simulink model "lane_keeping_MPC"  (R2020a)
settings: Solver=FixedStepAuto  StartTime=0.0  StopTime=13  FixedStep=.01  RelTol=1e-3
libraries: simulink x2, mpcadaslib x1
settings Model: EnablePacing=on  Creator=Jamie  LastModifiedBy=Jamie

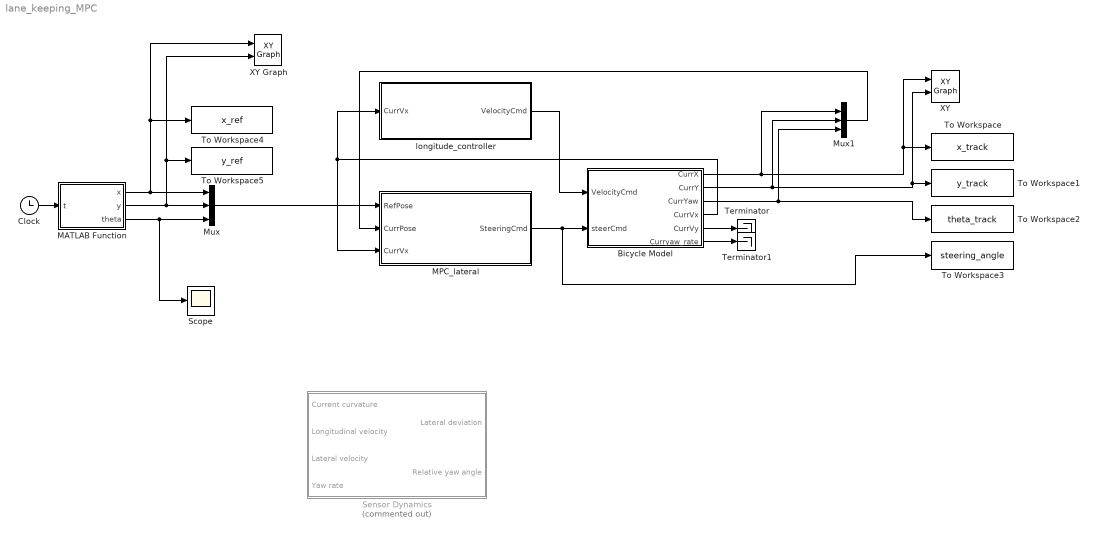
== system lane_keeping_MPC ==
  Bicycle Model : Subsystem
  Clock : Clock
  MATLAB Function : MATLAB Function  TreatAsAtomicUnit=on
  MPC_lateral : Subsystem
  Mux : Mux  Inputs=3
  Mux1 : Mux  Inputs=3
  Scope : Scope
  Sensor Dynamics : Subsystem  Commented=on
  Terminator : Terminator
  Terminator1 : Terminator
  To Workspace : ToWorkspace  VariableName=x_track  SampleTime=-1
      settings: Save2DSignal=2-D array (concatenate along first dimension)
  To Workspace1 : ToWorkspace  VariableName=y_track  SampleTime=-1
      settings: Save2DSignal=2-D array (concatenate along first dimension)
  To Workspace2 : ToWorkspace  VariableName=theta_track  SampleTime=-1
      settings: Save2DSignal=2-D array (concatenate along first dimension)
  To Workspace3 : ToWorkspace  VariableName=steering_angle  SampleTime=-1
      settings: Save2DSignal=2-D array (concatenate along first dimension)
  To Workspace4 : ToWorkspace  VariableName=x_ref  SampleTime=-1
      settings: Save2DSignal=2-D array (concatenate along first dimension)
  To Workspace5 : ToWorkspace  VariableName=y_ref  SampleTime=-1
      settings: Save2DSignal=2-D array (concatenate along first dimension)
  XY : simulink/Sinks/XY Graph  xmin=-10  xmax=10  ymin=-5  ymax=5  st=-1
  XY Graph : simulink/Sinks/XY Graph  xmin=-1  xmax=1  ymin=-1  ymax=1  st=-1
  longitude_controller : Subsystem
  wires:
  Clock/1 -> MATLAB Function/1(t)
  MATLAB Function/1(x) -> Mux/1, XY Graph/1, To Workspace4/1
  MATLAB Function/2(y) -> XY Graph/2, To Workspace5/1, Mux/2
  MATLAB Function/3(theta) -> Scope/1, Mux/3
  MPC_lateral/1(SteeringCmd) -> To Workspace3/1, Bicycle Model/2(steerCmd)
  Bicycle Model/3(CurrYaw) -> To Workspace2/1, Mux1/3
  Bicycle Model/1(CurrX) -> XY/1, To Workspace/1, Mux1/1
  Bicycle Model/2(CurrY) -> XY/2, To Workspace1/1, Mux1/2
  Mux1/1 -> MPC_lateral/2(CurrPose)
  Mux/1 -> MPC_lateral/1(RefPose)
  longitude_controller/1(VelocityCmd) -> Bicycle Model/1(VelocityCmd)
  Bicycle Model/4(CurrVx) -> MPC_lateral/3(CurrVx), longitude_controller/1(CurrVx)
  Bicycle Model/5(CurrVy) -> Terminator/1
  Bicycle Model/6(Curryaw_rate) -> Terminator1/1

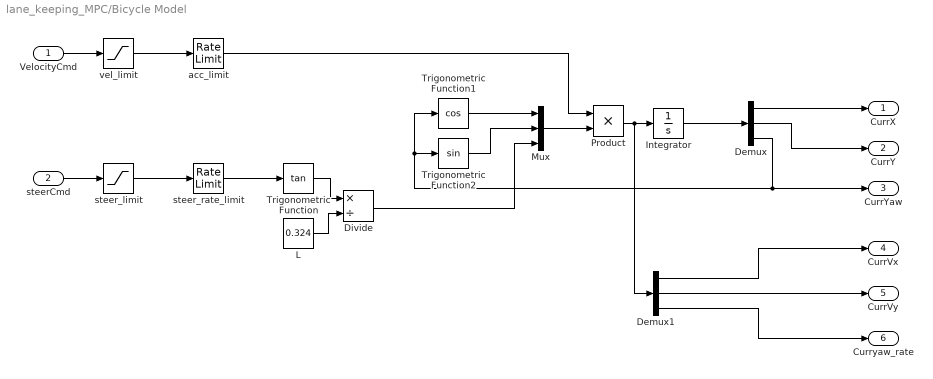
== system lane_keeping_MPC/Bicycle Model ==
  VelocityCmd : Inport
  steerCmd : Inport  Port=2
  Demux : Demux  Outputs=3
  Demux1 : Demux  Outputs=3
  Divide : Product  Inputs=*/
  Integrator : Integrator  InitialCondition=[0, 0, pi/2]
  L : Constant  Value=0.324
  Mux : Mux  Inputs=3
  Product : Product
  Trigonometric Function : Trigonometry  Operator=tan
  Trigonometric Function1 : Trigonometry  Operator=cos
  Trigonometric Function2 : Trigonometry
  acc_limit : RateLimiter  SampleTimeMode=inherited
  steer_limit : Saturate
  steer_rate_limit : RateLimiter  RisingSlewLimit=3  FallingSlewLimit=-3  SampleTimeMode=inherited
  vel_limit : Saturate  UpperLimit=3  LowerLimit=-3
  CurrX : Outport
  CurrY : Outport  Port=2
  CurrYaw : Outport  Port=3
  CurrVx : Outport  Port=4
  CurrVy : Outport  Port=5
  Curryaw_rate : Outport  Port=6
  wires:
  steerCmd/1 -> steer_limit/1
  VelocityCmd/1 -> vel_limit/1
  vel_limit/1 -> acc_limit/1
  steer_limit/1 -> steer_rate_limit/1
  steer_rate_limit/1 -> Trigonometric Function/1
  Trigonometric Function/1 -> Divide/1
  L/1 -> Divide/2
  acc_limit/1 -> Product/1
  Trigonometric Function1/1 -> Mux/1
  Trigonometric Function2/1 -> Mux/2
  Mux/1 -> Product/2
  Product/1 -> Demux1/1, Integrator/1
  Divide/1 -> Mux/3
  Integrator/1 -> Demux/1
  Demux/1 -> CurrX/1
  Demux/2 -> CurrY/1
  Demux/3 -> Trigonometric Function1/1, Trigonometric Function2/1, CurrYaw/1
  Demux1/1 -> CurrVx/1
  Demux1/2 -> CurrVy/1
  Demux1/3 -> Curryaw_rate/1

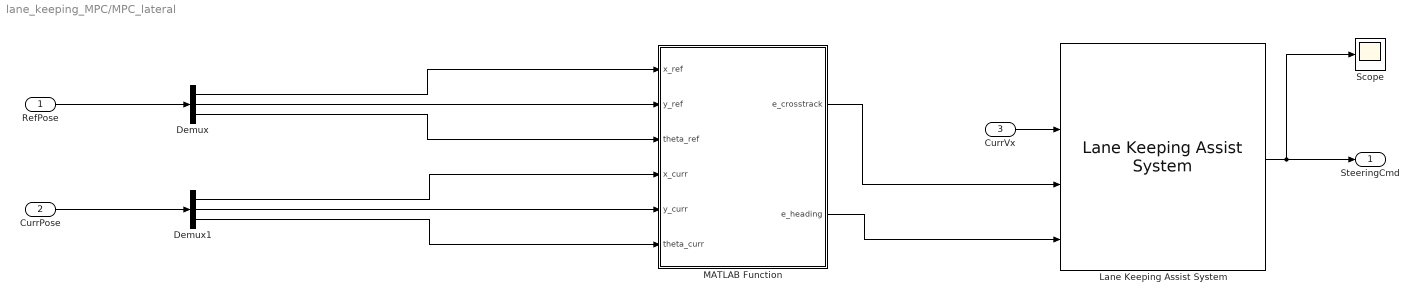
== system lane_keeping_MPC/MPC_lateral ==
  RefPose : Inport
  CurrPose : Inport  Port=2
  CurrVx : Inport  Port=3
  Demux : Demux  Outputs=3
  Demux1 : Demux  Outputs=3
  Lane Keeping Assist System : mpcadaslib/Lane Keeping Assist System  ModelType=Use vehicle parameters  VehicleMass=1575  VehicleYawInertia=2875  LengthToFront=1.2  LengthToRear=1.6  FrontTireStiffness=19000  RearTireStiffness=33000  EgoModelMatrixA=[-4.4021 ,-12.4603;1.3913,-5.1868]  EgoModelMatrixB=[24.1270;15.8609]  EgoModelMatrixC=[1,0;0,1]  InitialLongVel=1  TransportLag=0  MinSteering=-0.5  umin_ext=off  MaxSteering=0.5  umax_ext=off  Ts=0.01  PredictionHorizon=10  ControllerBehavior=1.0  suboptimal=off  maxiter=10  datatypeopt=double  optmode=off  trackmode=off
      settings: SourceProductBaseCode=MP
  MATLAB Function : MATLAB Function  TreatAsAtomicUnit=on
  Scope : Scope
  SteeringCmd : Outport
  wires:
  Demux/1 -> MATLAB Function/1(x_ref)
  Demux/2 -> MATLAB Function/2(y_ref)
  Demux/3 -> MATLAB Function/3(theta_ref)
  Demux1/1 -> MATLAB Function/4(x_curr)
  Demux1/2 -> MATLAB Function/5(y_curr)
  Demux1/3 -> MATLAB Function/6(theta_curr)
  Lane Keeping Assist System/1 -> Scope/1, SteeringCmd/1
  MATLAB Function/2(e_heading) -> Lane Keeping Assist System/4
  MATLAB Function/1(e_crosstrack) -> Lane Keeping Assist System/3
  CurrPose/1 -> Demux1/1
  RefPose/1 -> Demux/1
  CurrVx/1 -> Lane Keeping Assist System/2

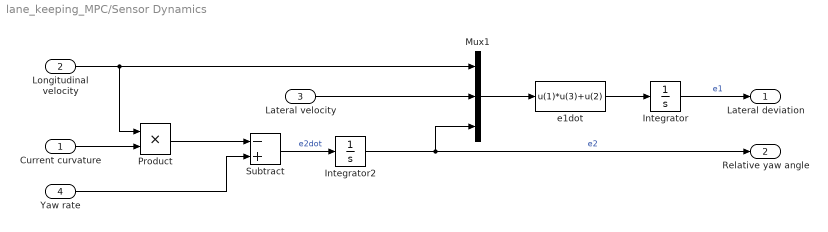
== system lane_keeping_MPC/Sensor Dynamics ==
  Current curvature : Inport
  Longitudinal velocity : Inport  Port=2
  Lateral velocity : Inport  Port=3
  Yaw rate : Inport  Port=4
  Integrator : Integrator
  Integrator2 : Integrator
  Mux1 : Mux  Inputs=[1 1 1]
  Product : Product
  Subtract : Sum  Inputs=-+
  e1dot : Fcn  Expr=u(1)*u(3)+u(2)
  Lateral deviation : Outport  VectorParamsAs1DForOutWhenUnconnected=off
  Relative yaw angle : Outport  Port=2  VectorParamsAs1DForOutWhenUnconnected=off
  wires:
  Current curvature/1 -> Product/2
  Integrator2/1 -> Mux1/3, Relative yaw angle/1  "e2"
  Mux1/1 -> e1dot/1
  e1dot/1 -> Integrator/1
  Longitudinal velocity/1 -> Product/1, Mux1/1
  Lateral velocity/1 -> Mux1/2
  Integrator/1 -> Lateral deviation/1  "e1"
  Product/1 -> Subtract/1
  Yaw rate/1 -> Subtract/2
  Subtract/1 -> Integrator2/1  "e2dot"

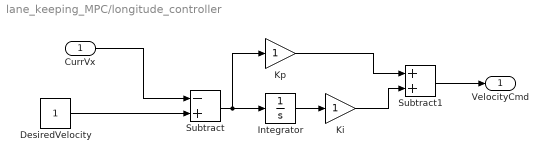
== system lane_keeping_MPC/longitude_controller ==
  CurrVx : Inport
  DesiredVelocity : Constant
  Integrator : Integrator  InitialCondition=0.001
  Ki : Gain
  Kp : Gain
  Subtract : Sum  Inputs=-+
  Subtract1 : Sum
  VelocityCmd : Outport
  wires:
  Subtract1/1 -> VelocityCmd/1
  DesiredVelocity/1 -> Subtract/2
  Ki/1 -> Subtract1/2
  Subtract/1 -> Integrator/1, Kp/1
  Integrator/1 -> Ki/1
  Kp/1 -> Subtract1/1
  CurrVx/1 -> Subtract/1

== matlab function lane_keeping_MPC/MPC_lateral/MATLAB Function ==
  data: x_ref input; e_crosstrack output; y_ref input; theta_ref input; x_curr input; y_curr input; theta_curr input; e_heading output
function [e_crosstrack, e_heading] = fcn(x_ref, y_ref, theta_ref, x_curr, y_curr, theta_curr)

e_crosstrack = x_curr*sin(theta_ref) - y_curr*cos(theta_ref) - x_ref*sin(theta_ref) + y_ref*cos(theta_ref);

e_heading =  theta_ref - theta_curr;

== matlab function lane_keeping_MPC/MATLAB Function ==
  data: t input; x output; y output; theta output
function [x, y, theta]= fcn(t)
pi = 3.14159;

v = 1;
R = 1;
T0 = pi*R/v;

if (t>4*T0)
    t = mod(t,(4*T0));
end
    
if ((t >= 0)&&(t <= 2*T0))
    x = R + R*cos(pi - (v/R)*t);
    y = R*sin(pi - (v/R)*t);
    theta = pi/2 - (v/R)*t;
elseif ((t >= 2*T0)&&(t <= 4*T0))
    x = -R - R*cos(pi + (v/R)*(-t + 2*T0));
    y = R*sin(pi + (v/R)*(-t + 2*T0));
    theta = -3*pi/2 + (v/R)*(t - 2*T0);
else 
    x = 0;
    y = 0;
    theta = pi/2;
end
